simulink model "engine_cl_tuned"  (R2020a)
settings: Solver=VariableStepAuto  StartTime=0  StopTime=options.T_train  MaxStep=0.01  RelTol=1e-3  EnableMultiTasking=on
PreLoadFcn:
  | Kp=0.0055;
  | Ki=0.0131;
  | Kd=3.3894e-004;
  | N=9.9135;
model workspace (MAT data in the model file):
  p = [-7.82997288351e-05; 0.181210895977; -0.072497134344; 0.000486358314052; 0.0361674637937]
undefined symbols (not defined in the file or in its folder): options
libraries: neural x92, simulink_need_slupdate x2, simulink x2
(part 4 of 5)

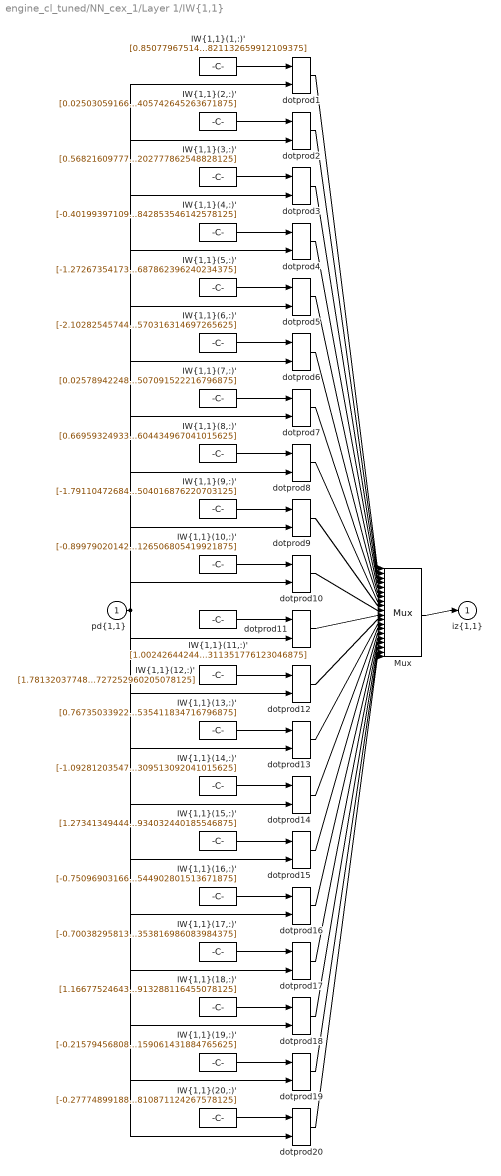
== system engine_cl_tuned/NN_cex_1/Layer 1/IW{1,1} ==
  "pd{1,1}" : Inport  PortDimensions=8
      mask Display: e = 0.06;c1 = [120 230 180]/255;c2 = ([120 230 180]+0)/(256+128);c3 = ([120 230 180]+128)/(256+128);patch([0 1 1 0],[0 0 1 1],c1);patch([0 1 1 1-e 1-e 0+e],[0 0 1 1-e 0+e 0+e],c2);patch([0 0 1 1-e 0+e 0+e],[0 1 1 1-e 1-e 0+e],c3);plot([0 1 1 0 0],[0 0 1 1 0]);
  "IW{1,1}(1,:)'" : Constant  Value=[0.85077967514548558103371078686905093491077423095703125;-0.22709479517275055204805767061770893633365631103515625;-1.09041708597097919408724919776432216167449951171875;1.176556194479629890992100627045147120952606201171875;-0.69885415809229878281172432252787984907627105712890625;0.269194515874013384770790935363038443028926849365234375;-0.1903177617019028711187189628617488779127597808837890625;0.393470258830906194358334460048354230821132659912109375]
      mask Display: e = 0.06;c1 = [120 150 230]/255;c2 = ([120 150 230]+0)/383;c3 = ([120 150 230]+128)/383;patch([0 1 1 0],[0 0 1 1],c1);patch([0 1 1 1-e 1-e 0+e],[0 0 1 1-e 0+e 0+e],c2);patch([0 0 1 1-e 0+e 0+e],[0 1 1 1-e 1-e 0+e],c3);plot([0 1 1 0 0],[0 0 1 1 0]);disp('Weights');
  "IW{1,1}(10,:)'" : Constant  Value=[-0.89979020142533361337200403795577585697174072265625;0.48402232350984453201903079389012418687343597412109375;0.77469694198627891967845471299369819462299346923828125;-1.132511034800044225079318493953905999660491943359375;-0.329862491198195717512220426215208135545253753662109375;-0.402536401604381255392439697970985434949398040771484375;-0.82935291619568707321974443402723409235477447509765625;-0.77065952964369877076222792311455123126506805419921875]
      mask Display: e = 0.06;c1 = [120 150 230]/255;c2 = ([120 150 230]+0)/383;c3 = ([120 150 230]+128)/383;patch([0 1 1 0],[0 0 1 1],c1);patch([0 1 1 1-e 1-e 0+e],[0 0 1 1-e 0+e 0+e],c2);patch([0 0 1 1-e 0+e 0+e],[0 1 1 1-e 1-e 0+e],c3);plot([0 1 1 0 0],[0 0 1 1 0]);disp('Weights');
  "IW{1,1}(11,:)'" : Constant  Value=[1.0024264424499929049261481850408017635345458984375;-0.212630436992708116150652131182141602039337158203125;-0.440618296050227564730761287137283943593502044677734375;-1.467355224460512364004216578905470669269561767578125;-1.9417946709122297921368272000108845531940460205078125;0.5514595431193265451241813934757374227046966552734375;0.0169279749352842408260944040421236422844231128692626953125;0.0260592356976700571802307848656710120849311351776123046875]
      mask Display: e = 0.06;c1 = [120 150 230]/255;c2 = ([120 150 230]+0)/383;c3 = ([120 150 230]+128)/383;patch([0 1 1 0],[0 0 1 1],c1);patch([0 1 1 1-e 1-e 0+e],[0 0 1 1-e 0+e 0+e],c2);patch([0 0 1 1-e 0+e 0+e],[0 1 1 1-e 1-e 0+e],c3);plot([0 1 1 0 0],[0 0 1 1 0]);disp('Weights');
  "IW{1,1}(12,:)'" : Constant  Value=[1.781320377480286598625980332144536077976226806640625;0.86031160586417743108000877327867783606052398681640625;0.946156989935427628068964622798375785350799560546875;1.1182801968230584588326337325270287692546844482421875;0.09043189127646357461376425135313184000551700592041015625;-0.05946028641874813447376624253593035973608493804931640625;-0.2337320947785384850359235997530049644410610198974609375;-1.0593596015514485930708588057314045727252960205078125]
      mask Display: e = 0.06;c1 = [120 150 230]/255;c2 = ([120 150 230]+0)/383;c3 = ([120 150 230]+128)/383;patch([0 1 1 0],[0 0 1 1],c1);patch([0 1 1 1-e 1-e 0+e],[0 0 1 1-e 0+e 0+e],c2);patch([0 0 1 1-e 0+e 0+e],[0 1 1 1-e 1-e 0+e],c3);plot([0 1 1 0 0],[0 0 1 1 0]);disp('Weights');
  "IW{1,1}(13,:)'" : Constant  Value=[0.7673503392216967089467516416334547102451324462890625;-0.84761956640450508704276444404968060553073883056640625;-0.319010252651223513709055623621679842472076416015625;0.8448722324611870337918162476853467524051666259765625;-0.2453455466749469848775078162361751310527324676513671875;0.07006503689649667965255730450735427439212799072265625;-0.9998935570655274052143113294732756912708282470703125;-0.63426365800214756784924929888802580535411834716796875]
      mask Display: e = 0.06;c1 = [120 150 230]/255;c2 = ([120 150 230]+0)/383;c3 = ([120 150 230]+128)/383;patch([0 1 1 0],[0 0 1 1],c1);patch([0 1 1 1-e 1-e 0+e],[0 0 1 1-e 0+e 0+e],c2);patch([0 0 1 1-e 0+e 0+e],[0 1 1 1-e 1-e 0+e],c3);plot([0 1 1 0 0],[0 0 1 1 0]);disp('Weights');
  "IW{1,1}(14,:)'" : Constant  Value=[-1.09281203547788852148414662224240601062774658203125;-0.82145949938328488570959962089546024799346923828125;-0.59996785021022558392900236867717467248439788818359375;-0.85596804094392109352185116222244687378406524658203125;-0.92183051553150752166487791328108869493007659912109375;-0.838101060099095018784964850055985152721405029296875;0.57643247036080336176411265114438720047473907470703125;0.003644367896995120460756911739963470608927309513092041015625]
      mask Display: e = 0.06;c1 = [120 150 230]/255;c2 = ([120 150 230]+0)/383;c3 = ([120 150 230]+128)/383;patch([0 1 1 0],[0 0 1 1],c1);patch([0 1 1 1-e 1-e 0+e],[0 0 1 1-e 0+e 0+e],c2);patch([0 0 1 1-e 0+e 0+e],[0 1 1 1-e 1-e 0+e],c3);plot([0 1 1 0 0],[0 0 1 1 0]);disp('Weights');
  "IW{1,1}(15,:)'" : Constant  Value=[1.2734134944412252021805898039019666612148284912109375;-0.906006580151114793153510618139989674091339111328125;0.2023363678703632151378855041912174783647060394287109375;0.8363392074568418710356354495161212980747222900390625;-2.193971720612661879812321785720996558666229248046875;0.38933862260895912843494670596555806696414947509765625;0.170153071835728975091939219055348075926303863525390625;-1.7358012318604731927251805245759896934032440185546875]
      mask Display: e = 0.06;c1 = [120 150 230]/255;c2 = ([120 150 230]+0)/383;c3 = ([120 150 230]+128)/383;patch([0 1 1 0],[0 0 1 1],c1);patch([0 1 1 1-e 1-e 0+e],[0 0 1 1-e 0+e 0+e],c2);patch([0 0 1 1-e 0+e 0+e],[0 1 1 1-e 1-e 0+e],c3);plot([0 1 1 0 0],[0 0 1 1 0]);disp('Weights');
  "IW{1,1}(16,:)'" : Constant  Value=[-0.75096903166254680428437495720572769641876220703125;0.9721619161939789588444682522094808518886566162109375;0.10833236456595986274553666817155317403376102447509765625;-0.6653209979558363240670360028161667287349700927734375;-1.4003323228555208945778076667920686304569244384765625;-0.9279747492041841017140768599347211420536041259765625;-0.74590611024837161213696390404948033392429351806640625;0.5686862636663760905975095738540403544902801513671875]
      mask Display: e = 0.06;c1 = [120 150 230]/255;c2 = ([120 150 230]+0)/383;c3 = ([120 150 230]+128)/383;patch([0 1 1 0],[0 0 1 1],c1);patch([0 1 1 1-e 1-e 0+e],[0 0 1 1-e 0+e 0+e],c2);patch([0 0 1 1-e 0+e 0+e],[0 1 1 1-e 1-e 0+e],c3);plot([0 1 1 0 0],[0 0 1 1 0]);disp('Weights');
  "IW{1,1}(17,:)'" : Constant  Value=[-0.7003829581364808820609368922305293381214141845703125;0.9141628657163101134841554085141979157924652099609375;-0.51702383093192849639052610655198805034160614013671875;1.5492927617291318842518421661225147545337677001953125;1.323968030676396789857562907855026423931121826171875;0.66338135644148799041630581996287219226360321044921875;-1.01038329560681550134404460550285875797271728515625;-0.442244902184798061028914162307046353816986083984375]
      mask Display: e = 0.06;c1 = [120 150 230]/255;c2 = ([120 150 230]+0)/383;c3 = ([120 150 230]+128)/383;patch([0 1 1 0],[0 0 1 1],c1);patch([0 1 1 1-e 1-e 0+e],[0 0 1 1-e 0+e 0+e],c2);patch([0 0 1 1-e 0+e 0+e],[0 1 1 1-e 1-e 0+e],c3);plot([0 1 1 0 0],[0 0 1 1 0]);disp('Weights');
  "IW{1,1}(18,:)'" : Constant  Value=[1.1667752464336675899403417133726179599761962890625;-0.114576385807654557158485886247945018112659454345703125;-0.75617174557694466496826635193428955972194671630859375;-0.7262985052001891261852506431750953197479248046875;0.1712455740111631652400348002629471011459827423095703125;0.7788602197037806096346912454464472830295562744140625;-0.56005535643161341585738455250975675880908966064453125;-0.474410838152344915830127547451411373913288116455078125]
      mask Display: e = 0.06;c1 = [120 150 230]/255;c2 = ([120 150 230]+0)/383;c3 = ([120 150 230]+128)/383;patch([0 1 1 0],[0 0 1 1],c1);patch([0 1 1 1-e 1-e 0+e],[0 0 1 1-e 0+e 0+e],c2);patch([0 0 1 1-e 0+e 0+e],[0 1 1 1-e 1-e 0+e],c3);plot([0 1 1 0 0],[0 0 1 1 0]);disp('Weights');
  "IW{1,1}(19,:)'" : Constant  Value=[-0.215794568088821192564097373178810812532901763916015625;-0.37688122856381289782490284778759814798831939697265625;0.04859095108187462541682322125780046917498111724853515625;-1.2935474048951187686640196261578239500522613525390625;1.42710606752627722215720496024005115032196044921875;0.93732893700476871412519130899454466998577117919921875;-0.73036472317535106046904047616408206522464752197265625;-0.79769969402808860170495108832255937159061431884765625]
      mask Display: e = 0.06;c1 = [120 150 230]/255;c2 = ([120 150 230]+0)/383;c3 = ([120 150 230]+128)/383;patch([0 1 1 0],[0 0 1 1],c1);patch([0 1 1 1-e 1-e 0+e],[0 0 1 1-e 0+e 0+e],c2);patch([0 0 1 1-e 0+e 0+e],[0 1 1 1-e 1-e 0+e],c3);plot([0 1 1 0 0],[0 0 1 1 0]);disp('Weights');
  "IW{1,1}(2,:)'" : Constant  Value=[0.0250305916695482445766263168707155273295938968658447265625;-0.3976875620413131695585207125986926257610321044921875;0.69718945506856144778140560447354800999164581298828125;0.76963157790640934763359837234020233154296875;0.96592082341238094667090763323358260095119476318359375;0.23129017110887328811941188178025186061859130859375;-1.0172353587819660258873000202584080398082733154296875;0.72824619261668999126158041690359823405742645263671875]
      mask Display: e = 0.06;c1 = [120 150 230]/255;c2 = ([120 150 230]+0)/383;c3 = ([120 150 230]+128)/383;patch([0 1 1 0],[0 0 1 1],c1);patch([0 1 1 1-e 1-e 0+e],[0 0 1 1-e 0+e 0+e],c2);patch([0 0 1 1-e 0+e 0+e],[0 1 1 1-e 1-e 0+e],c3);plot([0 1 1 0 0],[0 0 1 1 0]);disp('Weights');
  "IW{1,1}(20,:)'" : Constant  Value=[-0.277748991884470275426366470128414221107959747314453125;-0.89317162713055520129046271904371678829193115234375;0.445847547745629402271561048110015690326690673828125;-0.0355264283480551668059632675067405216395854949951171875;0.413179352578604996981681551915244199335575103759765625;-1.2418917068619872434709350272896699607372283935546875;0.9575457455047047261587067623622715473175048828125;-0.6724544104421348311717565593426115810871124267578125]
      mask Display: e = 0.06;c1 = [120 150 230]/255;c2 = ([120 150 230]+0)/383;c3 = ([120 150 230]+128)/383;patch([0 1 1 0],[0 0 1 1],c1);patch([0 1 1 1-e 1-e 0+e],[0 0 1 1-e 0+e 0+e],c2);patch([0 0 1 1-e 0+e 0+e],[0 1 1 1-e 1-e 0+e],c3);plot([0 1 1 0 0],[0 0 1 1 0]);disp('Weights');
  "IW{1,1}(3,:)'" : Constant  Value=[0.5682160977762709119787132294732145965099334716796875;0.94103822755900468077783216358511708676815032958984375;-0.87025002643858628825768164460896514356136322021484375;-0.8238991870388068239350332078174687922000885009765625;0.317851046237291157137150321432272903621196746826171875;-0.0303293912852747038488843145387363620102405548095703125;-0.806021383298525240235221644979901611804962158203125;-0.84899168012682324491180452241678722202777862548828125]
      mask Display: e = 0.06;c1 = [120 150 230]/255;c2 = ([120 150 230]+0)/383;c3 = ([120 150 230]+128)/383;patch([0 1 1 0],[0 0 1 1],c1);patch([0 1 1 1-e 1-e 0+e],[0 0 1 1-e 0+e 0+e],c2);patch([0 0 1 1-e 0+e 0+e],[0 1 1 1-e 1-e 0+e],c3);plot([0 1 1 0 0],[0 0 1 1 0]);disp('Weights');
  "IW{1,1}(4,:)'" : Constant  Value=[-0.401993971097662938785077813008683733642101287841796875;-0.65428586772778751790013984646066091954708099365234375;0.90372000444448497002980502657010219991207122802734375;-0.1263697909274829334069778496996150352060794830322265625;0.38771218047512479021321496475138701498508453369140625;-0.88138887738301707752697211617487482726573944091796875;0.9771871369700171339189864738727919757366180419921875;-0.6753093342415958932889452626113779842853546142578125]
      mask Display: e = 0.06;c1 = [120 150 230]/255;c2 = ([120 150 230]+0)/383;c3 = ([120 150 230]+128)/383;patch([0 1 1 0],[0 0 1 1],c1);patch([0 1 1 1-e 1-e 0+e],[0 0 1 1-e 0+e 0+e],c2);patch([0 0 1 1-e 0+e 0+e],[0 1 1 1-e 1-e 0+e],c3);plot([0 1 1 0 0],[0 0 1 1 0]);disp('Weights');
  "IW{1,1}(5,:)'" : Constant  Value=[-1.272673541730575674790770790423266589641571044921875;-0.53041120822966136838516604257165454328060150146484375;-0.65197739613060701202584823477081954479217529296875;0.11280146948146106689048195903524174354970455169677734375;0.4424438041217564343554613515152595937252044677734375;0.95621455981436387361327433609403669834136962890625;0.887606117916509784748768652207218110561370849609375;0.49575752824274965657735947388573549687862396240234375]
      mask Display: e = 0.06;c1 = [120 150 230]/255;c2 = ([120 150 230]+0)/383;c3 = ([120 150 230]+128)/383;patch([0 1 1 0],[0 0 1 1],c1);patch([0 1 1 1-e 1-e 0+e],[0 0 1 1-e 0+e 0+e],c2);patch([0 0 1 1-e 0+e 0+e],[0 1 1 1-e 1-e 0+e],c3);plot([0 1 1 0 0],[0 0 1 1 0]);disp('Weights');
  "IW{1,1}(6,:)'" : Constant  Value=[-2.102825457441639400713029317557811737060546875;-1.48375928486222630198199112783186137676239013671875;-0.43712855198629452235792314240825362503528594970703125;-0.0069690077999207573899997925082061556167900562286376953125;2.045291946110723291241129118134267628192901611328125;0.129286208859732021370092525103245861828327178955078125;-0.000506213386521721787729422015189584271865896880626678466796875;0.78593642812743758074844890870735980570316314697265625]
      mask Display: e = 0.06;c1 = [120 150 230]/255;c2 = ([120 150 230]+0)/383;c3 = ([120 150 230]+128)/383;patch([0 1 1 0],[0 0 1 1],c1);patch([0 1 1 1-e 1-e 0+e],[0 0 1 1-e 0+e 0+e],c2);patch([0 0 1 1-e 0+e 0+e],[0 1 1 1-e 1-e 0+e],c3);plot([0 1 1 0 0],[0 0 1 1 0]);disp('Weights');
  "IW{1,1}(7,:)'" : Constant  Value=[0.025789422487589981625166757339684409089386463165283203125;0.44235025169871822203759847980109043419361114501953125;-1.02513458844221982957378713763318955898284912109375;0.61686554381131297741802654854836873710155487060546875;0.14625826063886726569052143531735055148601531982421875;0.2154628064384067342995621174850384704768657684326171875;1.3911075939370274312523179105482995510101318359375;-0.727490199867151243751095535117201507091522216796875]
      mask Display: e = 0.06;c1 = [120 150 230]/255;c2 = ([120 150 230]+0)/383;c3 = ([120 150 230]+128)/383;patch([0 1 1 0],[0 0 1 1],c1);patch([0 1 1 1-e 1-e 0+e],[0 0 1 1-e 0+e 0+e],c2);patch([0 0 1 1-e 0+e 0+e],[0 1 1 1-e 1-e 0+e],c3);plot([0 1 1 0 0],[0 0 1 1 0]);disp('Weights');
  "IW{1,1}(8,:)'" : Constant  Value=[0.66959324933157271519945652471506036818027496337890625;-0.71080990554233647316095812129788100719451904296875;0.41737052942587771209304037256515584886074066162109375;-0.3772061975599110272838743185275234282016754150390625;-0.86394331347130870479844588771811686456203460693359375;-0.79429248817490638590044227385078556835651397705078125;1.136053249363544903616229930776171386241912841796875;-0.51733508492739643802593718646676279604434967041015625]
      mask Display: e = 0.06;c1 = [120 150 230]/255;c2 = ([120 150 230]+0)/383;c3 = ([120 150 230]+128)/383;patch([0 1 1 0],[0 0 1 1],c1);patch([0 1 1 1-e 1-e 0+e],[0 0 1 1-e 0+e 0+e],c2);patch([0 0 1 1-e 0+e 0+e],[0 1 1 1-e 1-e 0+e],c3);plot([0 1 1 0 0],[0 0 1 1 0]);disp('Weights');
  "IW{1,1}(9,:)'" : Constant  Value=[-1.7911047268439934665451573891914449632167816162109375;0.341468030705193548168807637921418063342571258544921875;0.7832490381180827743179406752460636198520660400390625;0.680673357266048828506654899683780968189239501953125;1.5882570908917419405526061382261104881763458251953125;-0.9033091323665127791997520034783519804477691650390625;-0.0428508120441979112325014966700109653174877166748046875;-1.1639663105738204951222769523155875504016876220703125]
      mask Display: e = 0.06;c1 = [120 150 230]/255;c2 = ([120 150 230]+0)/383;c3 = ([120 150 230]+128)/383;patch([0 1 1 0],[0 0 1 1],c1);patch([0 1 1 1-e 1-e 0+e],[0 0 1 1-e 0+e 0+e],c2);patch([0 0 1 1-e 0+e 0+e],[0 1 1 1-e 1-e 0+e],c3);plot([0 1 1 0 0],[0 0 1 1 0]);disp('Weights');
  Mux : Mux  Inputs=20
      mask Display: e = 0.06;c1 = [120 150 230]/255;c2 = ([120 150 230]+0)/383;c3 = ([120 150 230]+128)/383;patch([0 1 1 0],[0 0 1 1],c1);patch([0 1 1 1-e 1-e 0+e],[0 0 1 1-e 0+e 0+e],c2);patch([0 0 1 1-e 0+e 0+e],[0 1 1 1-e 1-e 0+e],c3);plot([0 1 1 0 0],[0 0 1 1 0]);disp('Mux');
  dotprod{1..20} (20 alike) : neural/Weight Functions/dotprod
  "iz{1,1}" : Outport
      mask Display: e = 0.06;c1 = [120 230 180]/255;c2 = ([120 230 180]+0)/(256+128);c3 = ([120 230 180]+128)/(256+128);patch([0 1 1 0],[0 0 1 1],c1);patch([0 1 1 1-e 1-e 0+e],[0 0 1 1-e 0+e 0+e],c2);patch([0 0 1 1-e 0+e 0+e],[0 1 1 1-e 1-e 0+e],c3);plot([0 1 1 0 0],[0 0 1 1 0]);
  wires:
  "IW{1,1}(1,:)'"/1 -> dotprod1/1
  "pd{1,1}"/1 -> dotprod1/2, dotprod2/2, dotprod3/2, dotprod4/2, dotprod5/2, dotprod6/2, dotprod7/2, dotprod8/2, dotprod9/2, dotprod10/2, dotprod11/2, dotprod12/2, dotprod13/2, dotprod14/2, dotprod15/2, dotprod16/2, dotprod17/2, dotprod18/2, dotprod19/2, dotprod20/2
  dotprod1/1 -> Mux/1
  "IW{1,1}(2,:)'"/1 -> dotprod2/1
  dotprod2/1 -> Mux/2
  "IW{1,1}(3,:)'"/1 -> dotprod3/1
  dotprod3/1 -> Mux/3
  "IW{1,1}(4,:)'"/1 -> dotprod4/1
  dotprod4/1 -> Mux/4
  "IW{1,1}(5,:)'"/1 -> dotprod5/1
  dotprod5/1 -> Mux/5
  "IW{1,1}(6,:)'"/1 -> dotprod6/1
  dotprod6/1 -> Mux/6
  "IW{1,1}(7,:)'"/1 -> dotprod7/1
  dotprod7/1 -> Mux/7
  "IW{1,1}(8,:)'"/1 -> dotprod8/1
  dotprod8/1 -> Mux/8
  "IW{1,1}(9,:)'"/1 -> dotprod9/1
  dotprod9/1 -> Mux/9
  "IW{1,1}(10,:)'"/1 -> dotprod10/1
  dotprod10/1 -> Mux/10
  "IW{1,1}(11,:)'"/1 -> dotprod11/1
  dotprod11/1 -> Mux/11
  "IW{1,1}(12,:)'"/1 -> dotprod12/1
  dotprod12/1 -> Mux/12
  "IW{1,1}(13,:)'"/1 -> dotprod13/1
  dotprod13/1 -> Mux/13
  "IW{1,1}(14,:)'"/1 -> dotprod14/1
  dotprod14/1 -> Mux/14
  "IW{1,1}(15,:)'"/1 -> dotprod15/1
  dotprod15/1 -> Mux/15
  "IW{1,1}(16,:)'"/1 -> dotprod16/1
  dotprod16/1 -> Mux/16
  "IW{1,1}(17,:)'"/1 -> dotprod17/1
  dotprod17/1 -> Mux/17
  "IW{1,1}(18,:)'"/1 -> dotprod18/1
  dotprod18/1 -> Mux/18
  "IW{1,1}(19,:)'"/1 -> dotprod19/1
  dotprod19/1 -> Mux/19
  "IW{1,1}(20,:)'"/1 -> dotprod20/1
  dotprod20/1 -> Mux/20
  Mux/1 -> "iz{1,1}"/1

== system engine_cl_tuned/NN_cex_1/Layer 2/Delays 1 ==
  "p{2}" : Inport  PortDimensions=20
      mask Display: e = 0.06;c1 = [120 230 180]/255;c2 = ([120 230 180]+0)/(256+128);c3 = ([120 230 180]+128)/(256+128);patch([0 1 1 0],[0 0 1 1],c1);patch([0 1 1 1-e 1-e 0+e],[0 0 1 1-e 0+e 0+e],c2);patch([0 0 1 1-e 0+e 0+e],[0 1 1 1-e 1-e 0+e],c3);plot([0 1 1 0 0],[0 0 1 1 0]);
  mux : Mux  Inputs=1
      mask Display: e = 0.06;c1 = [120 150 230]/255;c2 = ([120 150 230]+0)/383;c3 = ([120 150 230]+128)/383;patch([0 1 1 0],[0 0 1 1],c1);patch([0 1 1 1-e 1-e 0+e],[0 0 1 1-e 0+e 0+e],c2);patch([0 0 1 1-e 0+e 0+e],[0 1 1 1-e 1-e 0+e],c3);plot([0 1 1 0 0],[0 0 1 1 0]);disp('Mux')
  "pd{2,1}" : Outport
      mask Display: e = 0.06;c1 = [120 230 180]/255;c2 = ([120 230 180]+0)/(256+128);c3 = ([120 230 180]+128)/(256+128);patch([0 1 1 0],[0 0 1 1],c1);patch([0 1 1 1-e 1-e 0+e],[0 0 1 1-e 0+e 0+e],c2);patch([0 0 1 1-e 0+e 0+e],[0 1 1 1-e 1-e 0+e],c3);plot([0 1 1 0 0],[0 0 1 1 0]);
  wires:
  "p{2}"/1 -> mux/1
  mux/1 -> "pd{2,1}"/1
